simulink model "simu"  (R2019b)
settings: Solver=VariableStepAuto  StartTime=0.0  StopTime=4  RelTol=1e-3
values from neighbouring files (symbols this model uses):
  acp = K.A    [multi_p1.m]    (also in multi_p1b.m)
  ag = [ ... (first row only)    [multi_p2.m]
  bcp = K.B    [multi_p1.m]    (also in multi_p1b.m)
  bg = [0     0 ... (first row only)    [multi_p2.m]
  ccp = K.C    [multi_p1.m]    (also in multi_p1b.m)
  cg = [0     1     0     0     0     0 ... (first row only)    [multi_p2.m]
  dcp = K.D    [multi_p1.m]    (also in multi_p1b.m)
  dg = [0     0 ... (first row only)    [multi_p2.m]
settings Model: Creator=wddn  LastModifiedBy=fang
settings DataIOCC: ReturnWorkspaceOutputs=off
settings DebuggingCC: ArithmeticOperatorsInVariantConditions=warning
settings SFSimCC: SimUseLocalCustomCode=off  CustomCodeUndefinedFunction=UseInterfaceOnly
settings RTWCC: RTWUseLocalCustomCode=off

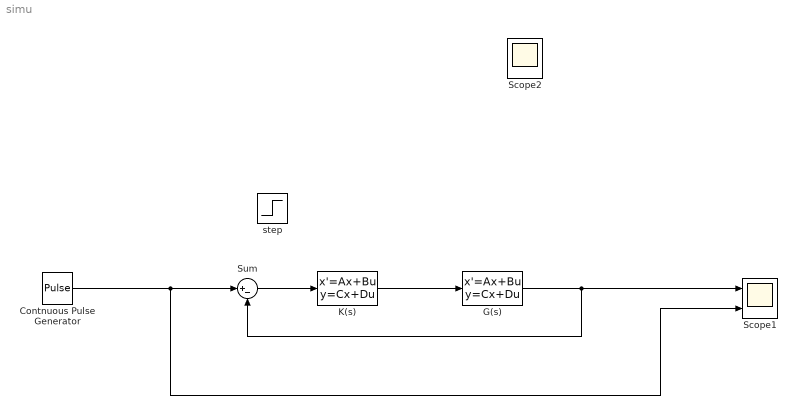
== system simu ==
  Contnuous Pulse Generator : DiscretePulseGenerator  PulseType=Time based  PulseWidth=50
  G(s) : StateSpace  A=ag  B=bg  C=cg  D=dg  InitialCondition=0
  K(s) : StateSpace  A=acp  B=bcp  C=ccp  D=dcp  InitialCondition=0
  Scope1 : Scope  NumInputPorts=2
  Scope2 : Scope  NumInputPorts=2
  Sum : Sum  Inputs=|+-
  step : Step  Time=0  SampleTime=0.1
  wires:
  G(s)/1 -> Scope1/1, Sum/2
  Sum/1 -> K(s)/1
  K(s)/1 -> G(s)/1
  Contnuous Pulse Generator/1 -> Scope1/2, Sum/1
